simulink model "lab7_FLC"  (R2020a)
settings: Solver=FixedStepAuto  StartTime=0.0  StopTime=400  FixedStep=0.01  RelTol=1e-3
values from neighbouring files (symbols this model uses):
  D = det(A)    [pplane8.m]
undefined symbols (not defined in the file or in its folder): g, h_bar, sigbuilder_block
libraries: simulink x1
settings Model: Creator=bruno  LastModifiedBy=bruno

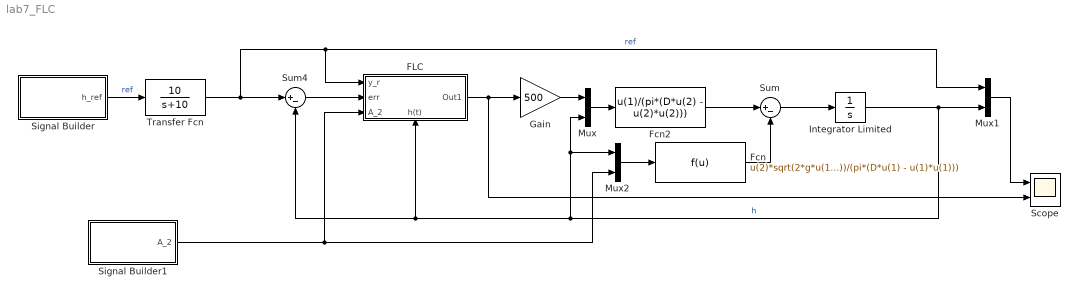
== system lab7_FLC ==
  FLC : Subsystem
      settings: PortSchema="{\"entries\":[{\"content\":{\"sides\":[{\"content\":{\"connectorIds\":[\"In1\",\"In2\",\"In3\"]},\"type\":\"ConnectorPlacement.EquallySpacedRectSide\",\"uuid\":\"da3e7f5a-9594-4c29-a0ec-3cc1ca63f264\"},{\"content\":{\"connectorIds\":[\"Out1\"],\"side\":\"RIGHT\"},\"type\":\"ConnectorPlacement.EquallySpacedRectSide\",\"uuid\":\"bdfa2608-d653-4e45-a46d-d46342907836\"},{\"content\":{\"connectorIds\":[],\"side\":\"TOP\"},\"type\":\"ConnectorPlacement.EquallySpacedRectSide\",\"uuid\":\"919ad7aa-dcde-46b6-9406-65efd00fdb72\"},{\"content\":{\"connectorIds\":[\"In4\"],\"side\":\"BOTTOM\"},\"type\":\"ConnectorPlacement.EquallySpacedRectSide\",\"uuid\":\"58c39bbf-f8fe-485d-a2fb-a32c56895a64\"}]},\"type\":\"ConnectorPlacement.EquallySpacedConnector\",\"uuid\":\"0132cd69-ef9c-4ff1-92b0-bdee72086be6\"}],\"packageUris\":[\"http://schema.mathworks.com/mf0/Connector/19700101\"],\"version\":\"1.0\"}"
  Fcn : Fcn  Expr=u(2)*sqrt(2*g*u(1))/(pi*(D*u(1) - u(1)*u(1)))
  Fcn2 : Fcn  Expr=u(1)/(pi*(D*u(2) - u(2)*u(2)))
  Gain : Gain  Gain=500
  Integrator Limited : Integrator  InitialCondition=h_bar  LimitOutput=on  UpperSaturationLimit=100-0.001  LowerSaturationLimit=0.001
  Mux : Mux  Inputs=2
  Mux1 : Mux  Inputs=2
  Mux2 : Mux  Inputs=2
  Scope : Scope  NumInputPorts=2
  Signal Builder : Subsystem  Tag=STV Subsys  LoadFcn=sigbuilder_block('load');  StartFcn=sigbuilder_block('start');  StopFcn=sigbuilder_block('stop');  ClipboardFcn=sigbuilder_block('clipboard');  mask(Sigbuilder block){tuvar=[0:10]}
      mask help: Simulink:masks:SigbuilderBlock_MD
      mask init:
      | if ~strcmp(get_param(bdroot(gcbh),'SimulationStatus'),'stopped') tuvar = sigbuilder_block('maskInit'); end
      settings: CopyFcn=sigbuilder_block('copy');  DeleteFcn=sigbuilder_block('delete');  ModelCloseFcn=sigbuilder_block('modelClose');  PreSaveFcn=sigbuilder_block('preSave');  PauseFcn=sigbuilder_block('pause');  ContinueFcn=sigbuilder_block('continue');  NameChangeFcn=sigbuilder_block('namechange');  OpenFcn=sigbuilder_block('open',[464.25 220.5 648 331.5 ]);  CloseFcn=sigbuilder_block('close');
      mask Display: plot(0, 0, 100, 100,[2, 2, 32, 32, 2], [68, 8, 8, 68, 68],[32, 2], [38, 38], [32, 19, 2],[53, 60, 44], [32, 17, 17, 2],[16, 16, 31, 31]);txt = getActiveGroup(gcbh);text(2, 100, txt,'verticalAlignment', 'top');
  Signal Builder1 : Subsystem  Tag=STV Subsys  LoadFcn=sigbuilder_block('load');  StartFcn=sigbuilder_block('start');  StopFcn=sigbuilder_block('stop');  ClipboardFcn=sigbuilder_block('clipboard');  mask(Sigbuilder block){tuvar=[0:10]}
      mask help: Simulink:masks:SigbuilderBlock_MD
      mask init:
      | if ~strcmp(get_param(bdroot(gcbh),'SimulationStatus'),'stopped') tuvar = sigbuilder_block('maskInit'); end
      settings: CopyFcn=sigbuilder_block('copy');  DeleteFcn=sigbuilder_block('delete');  ModelCloseFcn=sigbuilder_block('modelClose');  PreSaveFcn=sigbuilder_block('preSave');  PauseFcn=sigbuilder_block('pause');  ContinueFcn=sigbuilder_block('continue');  NameChangeFcn=sigbuilder_block('namechange');  OpenFcn=sigbuilder_block('open',[701.25 224.25 655.5 326.25 ]);  CloseFcn=sigbuilder_block('close');
      mask Display: plot(0, 0, 100, 100,[2, 2, 32, 32, 2], [68, 8, 8, 68, 68],[32, 2], [38, 38], [32, 19, 2],[53, 60, 44], [32, 17, 17, 2],[16, 16, 31, 31]);txt = getActiveGroup(gcbh);text(2, 100, txt,'verticalAlignment', 'top');
  Sum : Sum  Inputs=|+-
  Sum4 : Sum  Inputs=|+-
  Transfer Fcn : TransferFcn  Numerator=[10]  Denominator=[1 10]
  wires:
  Sum/1 -> Integrator Limited/1
  Fcn2/1 -> Sum/1
  Fcn/1 -> Sum/2
  Integrator Limited/1 -> Mux1/2, Mux2/1, Mux/2, FLC/4(h(t)), Sum4/2  "h"
  Transfer Fcn/1 -> Mux1/1, FLC/1(y_r), Sum4/1  "ref"
  Gain/1 -> Mux/1
  Mux/1 -> Fcn2/1
  Mux1/1 -> Scope/1
  Signal Builder1/1(A_2) -> FLC/3(A_2), Mux2/2
  FLC/1(Out1) -> Scope/2, Gain/1
  Sum4/1 -> FLC/2(err)
  Signal Builder/1(h_ref) -> Transfer Fcn/1  "ref"
  Mux2/1 -> Fcn/1

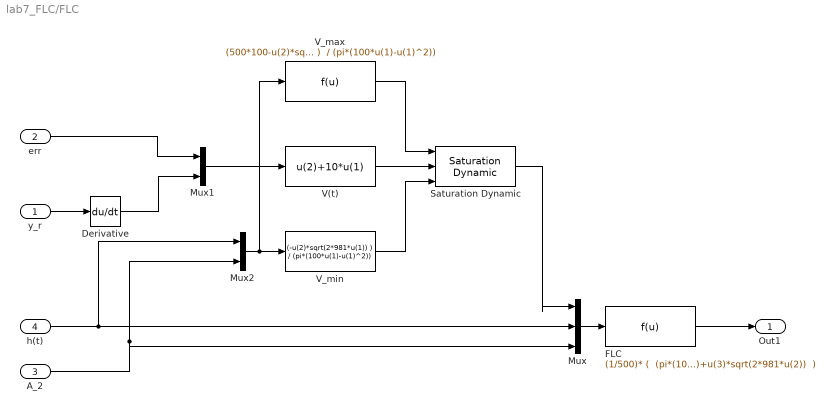
== system lab7_FLC/FLC ==
  y_r : Inport
  err : Inport  Port=2
  A_2 : Inport  Port=3
  h(t) : Inport  Port=4
  Derivative : Derivative
  FLC : Fcn  Expr="(1/500)* (  (pi*(100*u(2)-u(2)^2)) *u(1)+u(3)*sqrt(2*981*u(2))  )"
  Mux : Mux  Inputs=3
  Mux1 : Mux  Inputs=2
  Mux2 : Mux  Inputs=2
  Saturation Dynamic : simulink/Discontinuities/Saturation Dynamic  OutMin=[]  OutMax=[]  OutDataTypeStr=Inherit: Same as second input  OutDataType=fixdt(1, 16)  OutScaling=2^-10  DoSatur=off
  V(t) : Fcn  Expr=u(2)+10*u(1)
  V_max : Fcn  Expr="(500*100-u(2)*sqrt(2*981*u(1)) )  / (pi*(100*u(1)-u(1)^2))"
  V_min : Fcn  Expr="(-u(2)*sqrt(2*981*u(1))  ) / (pi*(100*u(1)-u(1)^2))"
  Out1 : Outport
  wires:
  FLC/1 -> Out1/1
  Mux/1 -> FLC/1
  A_2/1 -> Mux/3, Mux2/2
  h(t)/1 -> Mux2/1, Mux/2
  Mux1/1 -> V(t)/1
  y_r/1 -> Derivative/1
  err/1 -> Mux1/1
  Derivative/1 -> Mux1/2
  V(t)/1 -> Saturation Dynamic/2
  V_max/1 -> Saturation Dynamic/1
  V_min/1 -> Saturation Dynamic/3
  Mux2/1 -> V_max/1, V_min/1
  Saturation Dynamic/1 -> Mux/1

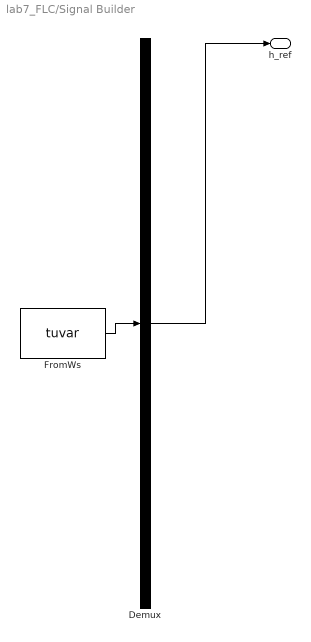
== system lab7_FLC/Signal Builder ==
  Demux : Demux  Tag=STV Demux  Outputs=1
      settings: DisplayOption=none
  FromWs : FromWorkspace  Tag=STV FromWs  VariableName=tuvar
      SigBuilderData=|
      | common.afterFinalStr = 'Extrapolate'
      | common.sampleTime = 0
      | dataSet.timeRange = [0 400]
      | dataSet.name = 'Group 1'
      | sbobj.Groups.Name = 'Group 1'
      | sbobj.Groups.Signals.Name = 'h_ref'
      | sbobj.Groups.Signals.XData = [0 50 50 150 150 250 250 300 300 400]
      | sbobj.Groups.Signals.YData = [90 90 50 50 10 10 50 50 90 90]
      | sbobj.Groups.TimeRange = [0 400]
  h_ref : Outport  Tag=STV Outport
  wires:
  Demux/1 -> h_ref/1
  FromWs/1 -> Demux/1

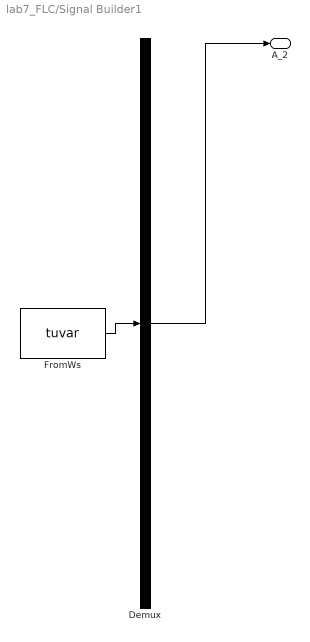
== system lab7_FLC/Signal Builder1 ==
  Demux : Demux  Tag=STV Demux  Outputs=1
      settings: DisplayOption=none
  FromWs : FromWorkspace  Tag=STV FromWs  VariableName=tuvar
      SigBuilderData=|
      | common.afterFinalStr = 'Extrapolate'
      | common.sampleTime = 0
      | dataSet.timeRange = [0 400]
      | dataSet.name = 'Group 1'
      | sbobj.Groups.Name = 'Group 1'
      | sbobj.Groups.Signals.Name = 'A_2'
      | sbobj.Groups.Signals.XData = [0 100 100 150 150 350 350 375 375 400]
      | sbobj.Groups.Signals.YData = [19.6 19.6 0 0 19.6 19.6 0 0 14.8 14.8]
      | sbobj.Groups.TimeRange = [0 400]
  A_2 : Outport  Tag=STV Outport
  wires:
  Demux/1 -> A_2/1
  FromWs/1 -> Demux/1
